simulink model "controller"  (R2025b)
settings: Solver=VariableStepAuto  StartTime=0.0  StopTime=inf  RelTol=1e-3
undefined symbols (not defined in the file): cog_height, DiscIntNeverNeededParam, Fz_stat_FL, Fz_stat_FR, Fz_stat_RL, Fz_stat_RR, lF, lR, pitch_inertia, pitchAngle, pitching_coefficient, pitchStiffness, rdyn, reference_area, rho, rollStiffness_F, rollStiffness_R, sprung_mass, tire, total_pitchDamping, total_pitchStiffness, total_rollStiffness, trackwidth_F, trackwidth_R, unsprung_mass, wheelbase
settings Model: Creator=marce  LastModifiedBy=marce

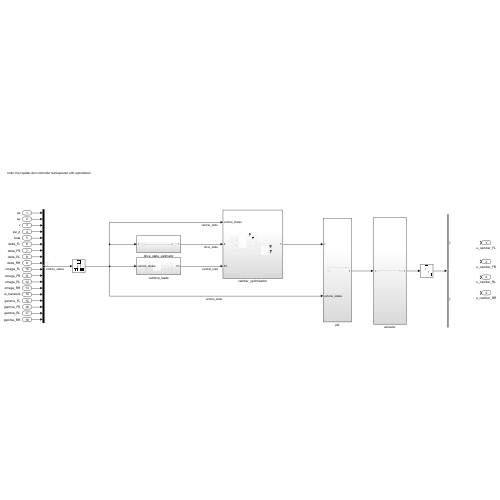
[thumbnail: Simulink's stored preview of the top-level diagram]
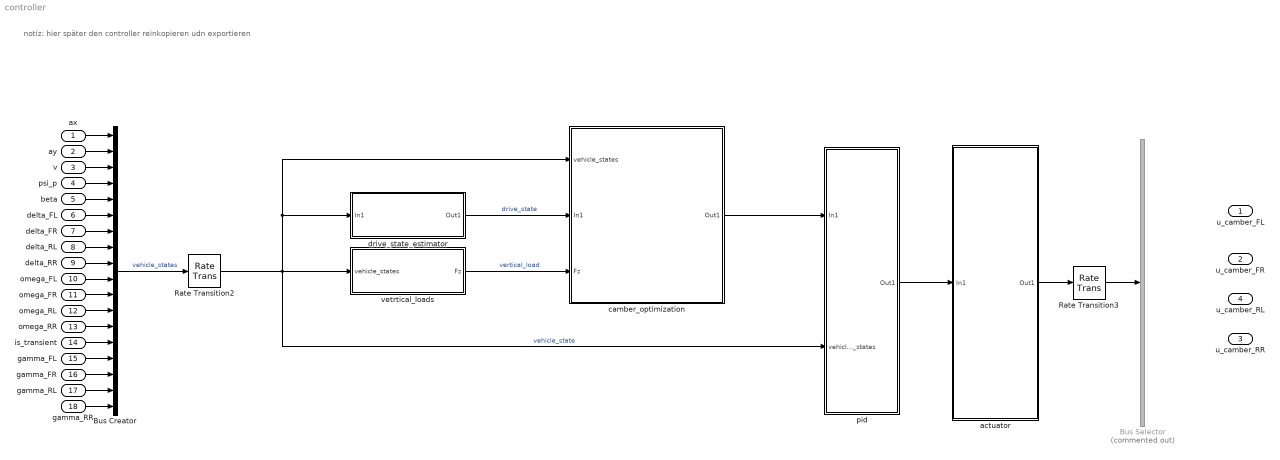
== system controller ==
  note: notiz: hier später den controller reinkopieren udn exportieren
  ax : Inport  OutDataTypeStr=double  Unit=m/s^2
  ay : Inport  Port=2  OutDataTypeStr=double  Unit=m/s^2
  v : Inport  Port=3  OutDataTypeStr=double  Unit=m/s
  psi_p : Inport  Port=4  OutDataTypeStr=double  Unit=rad/s
  beta : Inport  Port=5  OutDataTypeStr=double  Unit=rad
  delta_FL : Inport  Port=6  OutDataTypeStr=double  Unit=rad
  delta_FR : Inport  Port=7  OutDataTypeStr=double  Unit=rad
  delta_RL : Inport  Port=8  OutDataTypeStr=double  Unit=rad
  delta_RR : Inport  Port=9  OutDataTypeStr=double  Unit=rad
  omega_FL : Inport  Port=10  OutDataTypeStr=double  Unit=rad/s
  omega_FR : Inport  Port=11  OutDataTypeStr=double  Unit=rad/s
  omega_RL : Inport  Port=12  OutDataTypeStr=double  Unit=rad/s
  omega_RR : Inport  Port=13  OutDataTypeStr=double  Unit=rad/s
  is_transient : Inport  Port=14  OutDataTypeStr=boolean  Unit=1
  gamma_FL : Inport  Port=15  OutDataTypeStr=double  Unit=rad
  gamma_FR : Inport  Port=16  OutDataTypeStr=double  Unit=rad
  gamma_RL : Inport  Port=17  OutDataTypeStr=double  Unit=rad
  gamma_RR : Inport  Port=18  OutDataTypeStr=double  Unit=rad
  Bus Creator : BusCreator  Inputs=18  OutDataTypeStr=Bus: vehicle_states  NonVirtualBus=on
      settings: InheritFromInputs=off
  Bus Selector : BusSelector  Commented=on  OutputSignals=signal1,signal2
  Rate Transition2 : RateTransition
  Rate Transition3 : RateTransition
  actuator : Subsystem
  camber_optimization : Subsystem
  drive_state_estimator : Subsystem
  pid : Subsystem
  vetrtical_loads : Subsystem
  u_camber_FL : Outport
  u_camber_FR : Outport  Port=2
  u_camber_RR : Outport  Port=3
  u_camber_RL : Outport  Port=4
  wires:
  camber_optimization/1(Out1) -> pid/1(In1)
  Rate Transition2/1 -> camber_optimization/1(vehicle_states), drive_state_estimator/1(In1), vetrtical_loads/1(vehicle_states), pid/2(vehicle_states)  "vehicle_state"
  Rate Transition3/1 -> Bus Selector/1
  pid/1(Out1) -> actuator/1(In1)
  Bus Creator/1 -> Rate Transition2/1  "vehicle_states"
  vetrtical_loads/1(Fz) -> camber_optimization/3(Fz)  "vertical_load"
  drive_state_estimator/1(Out1) -> camber_optimization/2(In1)  "drive_state"
  actuator/1(Out1) -> Rate Transition3/1
  ax/1 -> Bus Creator/1
  ay/1 -> Bus Creator/2
  v/1 -> Bus Creator/3
  psi_p/1 -> Bus Creator/4
  beta/1 -> Bus Creator/5
  delta_FL/1 -> Bus Creator/6
  delta_FR/1 -> Bus Creator/7
  delta_RL/1 -> Bus Creator/8
  delta_RR/1 -> Bus Creator/9
  omega_FL/1 -> Bus Creator/10
  omega_FR/1 -> Bus Creator/11
  omega_RL/1 -> Bus Creator/12
  omega_RR/1 -> Bus Creator/13
  is_transient/1 -> Bus Creator/14
  gamma_FL/1 -> Bus Creator/15
  gamma_FR/1 -> Bus Creator/16
  gamma_RL/1 -> Bus Creator/17
  gamma_RR/1 -> Bus Creator/18

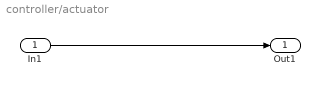
== system controller/actuator ==
  In1 : Inport
  Out1 : Outport
  wires:
  In1/1 -> Out1/1

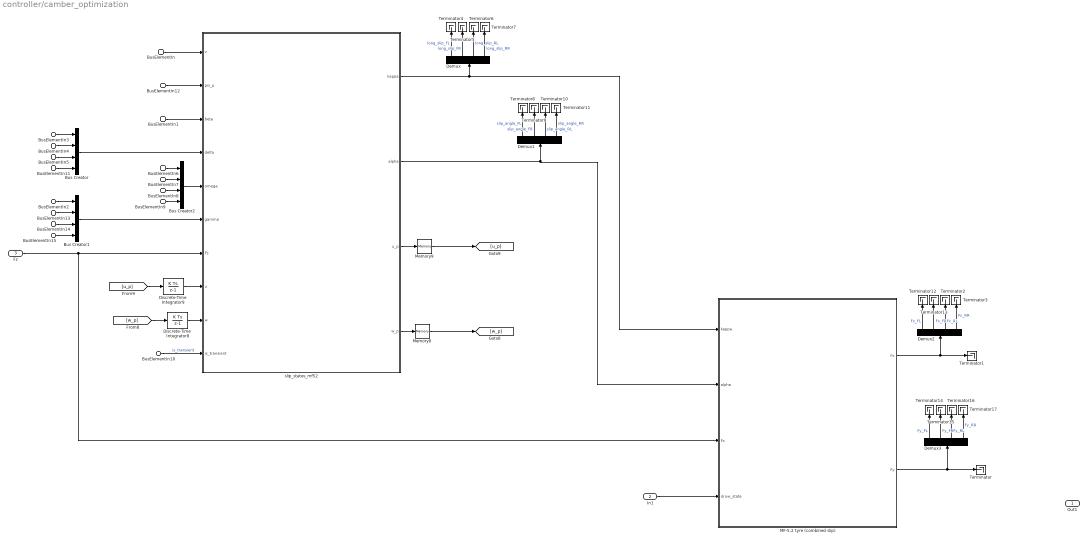
== system controller/camber_optimization ==
  BusElementIn6 : Inport  PortName=vehicle_states  Element=omega_FL
  BusElementIn7 : Inport  PortName=vehicle_states  Element=omega_FR
  BusElementIn8 : Inport  PortName=vehicle_states  Element=omega_RL
  BusElementIn9 : Inport  PortName=vehicle_states  Element=omega_RR
  BusElementIn10 : Inport  PortName=vehicle_states  Element=is_transient
  BusElementIn : Inport  PortName=vehicle_states  Element=v
  BusElementIn3 : Inport  PortName=vehicle_states  Element=delta_FL
  BusElementIn4 : Inport  PortName=vehicle_states  Element=delta_FR
  BusElementIn5 : Inport  PortName=vehicle_states  Element=delta_RL
  BusElementIn11 : Inport  PortName=vehicle_states  Element=delta_RR
  BusElementIn12 : Inport  PortName=vehicle_states  Element=yaw_rate
  BusElementIn1 : Inport  PortName=vehicle_states  Element=side_slip_angle
  BusElementIn2 : Inport  PortName=vehicle_states  Element=camber_FL
  BusElementIn13 : Inport  PortName=vehicle_states  Element=camber_FR
  BusElementIn14 : Inport  PortName=vehicle_states  Element=camber_RL
  BusElementIn15 : Inport  PortName=vehicle_states  Element=camber_RR
  In1 : Inport  Port=2
  Fz : Inport  Port=3
  Bus Creator : BusCreator  Inputs=4
  Bus Creator1 : BusCreator  Inputs=4
  Bus Creator2 : BusCreator  Inputs=4
  Demux{,1..3} (4 alike) : Demux
      settings: DisplayOption=none
  Discrete-Time Integrator8 : DiscreteIntegrator  SampleTime=-1  UpperSaturationLimit=0.1  LowerSaturationLimit=-0.1  ICPrevOutput=DiscIntNeverNeededParam  ICPrevScaledInput=DiscIntNeverNeededParam
  Discrete-Time Integrator9 : DiscreteIntegrator  SampleTime=-1  UpperSaturationLimit=0.01  LowerSaturationLimit=-0.01  ICPrevOutput=DiscIntNeverNeededParam  ICPrevScaledInput=DiscIntNeverNeededParam
  MF-5.2 tyre (combined slip) : MATLAB Function  TreatAsAtomicUnit=on
  Memory8 : Memory
  Memory9 : Memory
  Terminator{,1..17} (18 alike) : Terminator
  slip_states_mf52 : MATLAB Function  TreatAsAtomicUnit=on
  Out1 : Outport
  wires:
  Fz/1 -> slip_states_mf52/7(Fz), MF-5.2 tyre (combined slip)/3(Fz)
  BusElementIn6/1 -> Bus Creator2/1
  BusElementIn7/1 -> Bus Creator2/2
  BusElementIn10/1 -> slip_states_mf52/10(is_transient)  "is_transient"
  BusElementIn8/1 -> Bus Creator2/3
  BusElementIn9/1 -> Bus Creator2/4
  BusElementIn3/1 -> Bus Creator/1
  BusElementIn11/1 -> Bus Creator/4
  BusElementIn5/1 -> Bus Creator/3
  BusElementIn4/1 -> Bus Creator/2
  Bus Creator/1 -> slip_states_mf52/4(delta)
  BusElementIn/1 -> slip_states_mf52/1(v)
  [w_p] -> Discrete-Time Integrator8/1
  Discrete-Time Integrator8/1 -> slip_states_mf52/9(w)
  slip_states_mf52/4(w_p) -> Memory8/1
  Memory8/1 -> [w_p]
  Memory9/1 -> [u_p]
  slip_states_mf52/3(u_p) -> Memory9/1
  [u_p] -> Discrete-Time Integrator9/1
  Discrete-Time Integrator9/1 -> slip_states_mf52/8(u)
  slip_states_mf52/1(kappa) -> MF-5.2 tyre (combined slip)/1(kappa), Demux/1
  slip_states_mf52/2(alpha) -> MF-5.2 tyre (combined slip)/2(alpha), Demux1/1
  BusElementIn12/1 -> slip_states_mf52/2(psi_p)
  BusElementIn1/1 -> slip_states_mf52/3(beta)
  Bus Creator2/1 -> slip_states_mf52/5(omega)
  Demux/1 -> Terminator4/1  "long_slip_FL"
  Demux/2 -> Terminator5/1  "long_slip_FR"
  Demux/3 -> Terminator6/1  "long_slip_RL"
  Demux/4 -> Terminator7/1  "long_slip_RR"
  Demux1/2 -> Terminator9/1  "slip_angle_FR"
  Demux1/1 -> Terminator8/1  "slip_angle_FL"
  Demux1/4 -> Terminator11/1  "slip_angle_RR"
  Demux1/3 -> Terminator10/1  "slip_angle_RL"
  In1/1 -> MF-5.2 tyre (combined slip)/4(drive_state)
  MF-5.2 tyre (combined slip)/1(Fx) -> Demux2/1, Terminator1/1
  MF-5.2 tyre (combined slip)/2(Fy) -> Demux3/1, Terminator/1
  Demux2/2 -> Terminator13/1  "Fx_FR"
  Demux2/4 -> Terminator3/1  "Fx_RR"
  Demux2/3 -> Terminator2/1  "Fx_RL"
  Demux2/1 -> Terminator12/1  "Fx_FL"
  Demux3/3 -> Terminator16/1  "Fy_RL"
  Demux3/4 -> Terminator17/1  "Fy_RR"
  Demux3/1 -> Terminator14/1  "Fy_FL"
  Demux3/2 -> Terminator15/1  "Fy_FR"
  Bus Creator1/1 -> slip_states_mf52/6(gamma)
  BusElementIn2/1 -> Bus Creator1/1
  BusElementIn13/1 -> Bus Creator1/2
  BusElementIn14/1 -> Bus Creator1/3
  BusElementIn15/1 -> Bus Creator1/4

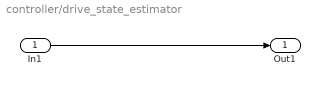
== system controller/drive_state_estimator ==
  In1 : Inport
  Out1 : Outport
  wires:
  In1/1 -> Out1/1

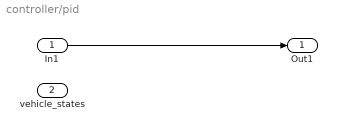
== system controller/pid ==
  In1 : Inport
  vehicle_states : Inport  Port=2
  Out1 : Outport
  wires:
  In1/1 -> Out1/1

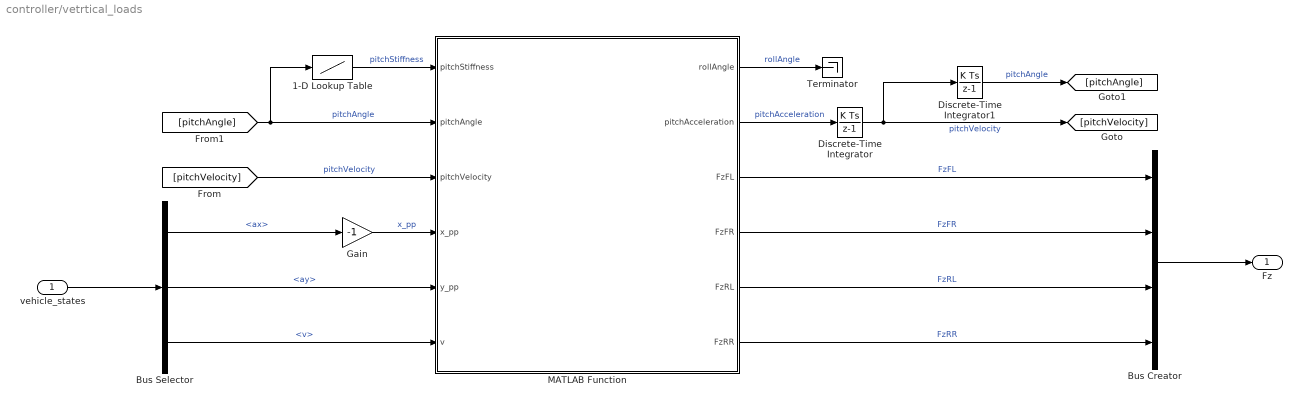
== system controller/vetrtical_loads ==
  vehicle_states : Inport
  1-D Lookup Table : Lookup_n-D  NumberOfTableDimensions=1  BreakpointsForDimension1=pitchAngle  Table=pitchStiffness  InternalRulePriority=Speed  RndMeth=Simplest
  Bus Creator : BusCreator  Inputs=4
  Bus Selector : BusSelector  OutputSignals=ax,ay,v
  Discrete-Time Integrator : DiscreteIntegrator  SampleTime=-1  ICPrevOutput=DiscIntNeverNeededParam  ICPrevScaledInput=DiscIntNeverNeededParam
  Discrete-Time Integrator1 : DiscreteIntegrator  InitialCondition=-0.001  SampleTime=-1  ICPrevOutput=DiscIntNeverNeededParam  ICPrevScaledInput=DiscIntNeverNeededParam
  Gain : Gain  Gain=-1
  MATLAB Function : MATLAB Function  TreatAsAtomicUnit=on
  Terminator : Terminator
  Fz : Outport
  wires:
  MATLAB Function/3(FzFL) -> Bus Creator/1  "FzFL"
  Discrete-Time Integrator1/1 -> [pitchAngle]  "pitchAngle"
  [pitchVelocity] -> MATLAB Function/3(pitchVelocity)  "pitchVelocity"
  Bus Selector/1 -> Gain/1  "<ax>"
  1-D Lookup Table/1 -> MATLAB Function/1(pitchStiffness)  "pitchStiffness"
  MATLAB Function/4(FzFR) -> Bus Creator/2  "FzFR"
  Gain/1 -> MATLAB Function/4(x_pp)  "x_pp"
  MATLAB Function/2(pitchAcceleration) -> Discrete-Time Integrator/1  "pitchAcceleration"
  [pitchAngle] -> 1-D Lookup Table/1, MATLAB Function/2(pitchAngle)  "pitchAngle"
  MATLAB Function/5(FzRL) -> Bus Creator/3  "FzRL"
  MATLAB Function/6(FzRR) -> Bus Creator/4  "FzRR"
  vehicle_states/1 -> Bus Selector/1
  Discrete-Time Integrator/1 -> [pitchVelocity], Discrete-Time Integrator1/1  "pitchVelocity"
  Bus Creator/1 -> Fz/1
  MATLAB Function/1(rollAngle) -> Terminator/1  "rollAngle"
  Bus Selector/2 -> MATLAB Function/5(y_pp)  "<ay>"
  Bus Selector/3 -> MATLAB Function/6(v)  "<v>"

== matlab function controller/vetrtical_loads/MATLAB Function ==
  data: pitchStiffness input; pitchAngle input; pitchVelocity input; x_pp input; rollAngle output; pitchAcceleration output; y_pp input; v input; cog_height parameter; sprung_mass parameter; FzFL output; rollStiffness_F parameter; rollStiffness_R parameter; total_rollStiffness parameter; trackwidth_F parameter; trackwidth_R parameter; Fz_stat_FL parameter; Fz_stat_FR parameter; Fz_stat_RL parameter; Fz_stat_RR parameter; FzFR output; FzRL output; FzRR output; wheelbase parameter; total_pitchStiffness parameter; rdyn parameter; unsprung_mass parameter; pitch_inertia parameter; total_pitchDamping parameter; reference_area parameter; pitching_coefficient parameter; rho parameter
function [rollAngle,pitchAcceleration,FzFL,FzFR,FzRL,FzRR]  = fcn(pitchStiffness,pitchAngle,pitchVelocity,x_pp, y_pp,v, cog_height, sprung_mass,rollStiffness_F,rollStiffness_R,total_rollStiffness,trackwidth_F, trackwidth_R, Fz_stat_FL, Fz_stat_FR, Fz_stat_RL, Fz_stat_RR, wheelbase, total_pitchStiffness, rdyn, unsprung_mass, pitch_inertia, total_pitchDamping, reference_area, pitching_coefficient, rho)

rollTorque = sprung_mass .* y_pp .* cog_height;
rollAngle = rollTorque ./ (total_rollStiffness);

dFz_roll_FL = (rollAngle .* rollStiffness_F - rdyn .* unsprung_mass .* y_pp) ./ trackwidth_F;
dFz_roll_FR = (rollAngle .* rollStiffness_F - rdyn .* unsprung_mass .* y_pp) ./ trackwidth_F;
dFz_roll_RL = (rollAngle .* rollStiffness_R - rdyn .* unsprung_mass .* y_pp) ./ trackwidth_R;
dFz_roll_RR = (rollAngle .* rollStiffness_R - rdyn .* unsprung_mass .* y_pp) ./ trackwidth_R;
           
pitchTorque = sprung_mass .* x_pp .* cog_height - rho ./2 .* pitching_coefficient .* wheelbase .* reference_area .* v^2;
% pitchStiffness = 3.825903e+09 * pitchAngle^3 + -1.854731e+09 * pitchAngle^2 + 1.728035e+08 * pitchAngle + -1.759672e+06;
% pitchStiffness = min(max(pitchStiffness, 290e3), 626e3);
pitchAcceleration = (pitchTorque - total_pitchDamping .* pitchVelocity - pitchStiffness .* pitchAngle) ./ pitch_inertia;

dFz_pitch_FL = (pitchStiffness ./ 2 .* pitchAngle + total_pitchDamping ./ 2 .* pitchVelocity - pitch_inertia ./4 .* pitchAcceleration) ./ wheelbase;
dFz_pitch_FR = (pitchStiffness ./ 2 .* pitchAngle + total_pitchDamping ./ 2 .* pitchVelocity - pitch_inertia ./4 .* pitchAcceleration) ./ wheelbase;
dFz_pitch_RL = (pitchStiffness ./ 2 .* pitchAngle + total_pitchDamping ./ 2 .* pitchVelocity - pitch_inertia ./4 .* pitchAcceleration) ./ wheelbase;
dFz_pitch_RR = (pitchStiffness ./ 2 .* pitchAngle + total_pitchDamping ./ 2 .* pitchVelocity - pitch_inertia ./4 .* pitchAcceleration) ./ wheelbase;

FzFL = Fz_stat_FL + dFz_roll_FL + dFz_pitch_FL;
FzFR = Fz_stat_FR - dFz_roll_FR + dFz_pitch_FR;
FzRL = Fz_stat_RL + dFz_roll_RL - dFz_pitch_RL;
FzRR = Fz_stat_RR - dFz_roll_RR - dFz_pitch_RR;

== matlab function controller/camber_optimization/MF-5.2 tyre (combined slip) ==
  data: kappa input; alpha input; Fz input; drive_state input; Fx output; tire parameter; Fy output
function [Fx, Fy] = fcn(kappa, alpha, Fz, drive_state, tire)
    %% determine output sizes
    % step is needed so simulink now the sizes when compiling
    Fx = zeros(1,4);
    Fy = zeros(1,4);

    %% camber
    gamma_FL = 0; % tyre model needs camber as input wich will be 0 for now
    gamma_FR = 0; % tyre model needs camber as input wich will be 0 for now
    gamma_RL = 0; % tyre model needs camber as input wich will be 0 for now
    gamma_RR = 0; % tyre model needs camber as input wich will be 0 for now

    %% parameter mapping
    % vertical
    F_z0 = tire.Vertical.FNOMIN;

    % longitudinal (pure slip)
    p_Cx1 = tire.Long.PCX1;
    
    p_Dx1 = tire.Long.PDX1;
    p_Dx2 = tire.Long.PDX2;
    p_Dx3 = tire.Long.PDX3;
    
    p_Ex1 = tire.Long.PEX1;
    p_Ex2 = tire.Long.PEX2;
    p_Ex3 = tire.Long.PEX3;
    p_Ex4 = tire.Long.PEX4;
    
    p_Kx1 = tire.Long.PKX1;
    p_Kx2 = tire.Long.PKX2;
    p_Kx3 = tire.Long.PKX3;
    
    p_Hx1 = tire.Long.PHX1;
    p_Hx2 = tire.Long.PHX2;
    
    p_Vx1 = tire.Long.PVX1;
    p_Vx2 = tire.Long.PVX2;
    
    % lateral (pure slip)
    p_Cy1 = tire.Lat.PCY1;
    
    p_Dy1 = tire.Lat.PDY1;
    p_Dy2 = tire.Lat.PDY2;
    p_Dy3 = tire.Lat.PDY3;
    
    p_Ey1 = tire.Lat.PEY1;
    p_Ey2 = tire.Lat.PEY2;
    p_Ey3 = tire.Lat.PEY3;
    p_Ey4 = tire.Lat.PEY4;
    
    p_Ky1 = tire.Lat.PKY1;
    p_Ky2 = tire.Lat.PKY2;
    p_Ky3 = tire.Lat.PKY3;
    
    p_Hy1 = tire.Lat.PHY1;
    p_Hy2 = tire.Lat.PHY2;
    p_Hy3 = tire.Lat.PHY3;
    
    p_Vy1 = tire.Lat.PVY1;
    p_Vy2 = tire.Lat.PVY2;
    p_Vy3 = tire.Lat.PVY3;
    p_Vy4 = tire.Lat.PVY4;
    
    % longitudinal (combined slip)
    r_Bx1 = tire.Long.RBX1;
    r_Bx2 = tire.Long.RBX2;
    
    r_Cx1 = tire.Long.RCX1;
    
    r_Ex1 = tire.Long.REX1;
    r_Ex2 = tire.Long.REX2;
    
    r_Hx1 = tire.Long.RHX1;
    
    % lateral (combined slip)
    r_By1 = tire.Lat.RBY1;
    r_By2 = tire.Lat.RBY2;
    r_By3 = tire.Lat.RBY3;
    
    r_Cy1 = tire.Lat.RCY1;
    
    r_Ey1 = tire.Lat.REY1;
    r_Ey2 = tire.Lat.REY2;
    
    r_Hy1 = tire.Lat.RHY1;
    r_Hy2 = tire.Lat.RHY2;
    
    r_Vy1 = tire.Lat.RVY1;
    r_Vy2 = tire.Lat.RVY2;
    r_Vy3 = tire.Lat.RVY3;
    r_Vy4 = tire.Lat.RVY4;
    r_Vy5 = tire.Lat.RVY5;
    r_Vy6 = tire.Lat.RVY6;

    %% vertical load mapping
    Fz_FL = Fz(1);
    Fz_FR = Fz(2);
    Fz_RL = Fz(3);
    Fz_RR = Fz(4);

    %% longitudinal slip mapping
    long_slip_FL = kappa(1);
    long_slip_FR = kappa(2);
    long_slip_RL = kappa(3);
    long_slip_RR = kappa(4);

    %% side slip angle mapping
    slip_ang_FL = alpha(1);
    slip_ang_FR = alpha(2);
    slip_ang_RL = alpha(3);
    slip_ang_RR = alpha(4);

    %% normalized vertical load
    % equations from Delft MF-Tyre User Manual Version 5.2
    % page 17
    dfz_FL = (Fz_FL - F_z0) / F_z0;
    dfz_FR = (Fz_FR - F_z0) / F_z0; 
    dfz_RL = (Fz_RL - F_z0) / F_z0; 
    dfz_RR = (Fz_RR - F_z0) / F_z0;

    %% longitudinal (pure slip)
    % equations from Delft MF-Tyre User Manual Version 5.2
    % page 22 - 24
    Cx = p_Cx1; % - each wheel is equipped with the same tyre
    
    mu_x_FL = (p_Dx1 + p_Dx2 .* dfz_FL) .* (1 - p_Dx3 .* gamma_FL.^2);
    mu_x_FR = (p_Dx1 + p_Dx2 .* dfz_FR) .* (1 - p_Dx3 .* gamma_FR.^2);
    mu_x_RL = (p_Dx1 + p_Dx2 .* dfz_RL) .* (1 - p_Dx3 .* gamma_RL.^2);
    mu_x_RR = (p_Dx1 + p_Dx2 .* dfz_RR) .* (1 - p_Dx3 .* gamma_RR.^2);

    Dx_FL = mu_x_FL .* Fz_FL;
    Dx_FR = mu_x_FR .* Fz_FR;
    Dx_RL = mu_x_RL .* Fz_RL;
    Dx_RR = mu_x_RR .* Fz_RR;
    
    S_Hx_FL = (p_Hx1 + p_Hx2 .* dfz_FL);
    S_Hx_FR = (p_Hx1 + p_Hx2 .* dfz_FR);
    S_Hx_RL = (p_Hx1 + p_Hx2 .* dfz_RL);
    S_Hx_RR = (p_Hx1 + p_Hx2 .* dfz_RR);

    S_Vx_FL = Fz_FL .* (p_Vx1 + p_Vx2 .* dfz_FL);
    S_Vx_FR = Fz_FR .* (p_Vx1 + p_Vx2 .* dfz_FR);
    S_Vx_RL = Fz_RL .* (p_Vx1 + p_Vx2 .* dfz_RL);
    S_Vx_RR = Fz_RR .* (p_Vx1 + p_Vx2 .* dfz_RR);
    
    kappa_x_FL = long_slip_FL + S_Hx_FL;
    kappa_x_FR = long_slip_FR + S_Hx_FR;
    kappa_x_RL = long_slip_RL + S_Hx_RL;
    kappa_x_RR = long_slip_RR + S_Hx_RR;
    
    Ex_FL = (p_Ex1 + p_Ex2 .* dfz_FL + p_Ex3 .* dfz_FL.^2) .* (1 - p_Ex4 .* sign(kappa_x_FL));
    Ex_FR = (p_Ex1 + p_Ex2 .* dfz_FR + p_Ex3 .* dfz_FR.^2) .* (1 - p_Ex4 .* sign(kappa_x_FR));
    Ex_RL = (p_Ex1 + p_Ex2 .* dfz_RL + p_Ex3 .* dfz_RL.^2) .* (1 - p_Ex4 .* sign(kappa_x_RL));
    Ex_RR = (p_Ex1 + p_Ex2 .* dfz_RR + p_Ex3 .* dfz_RR.^2) .* (1 - p_Ex4 .* sign(kappa_x_RR));

    Kx_FL = Fz_FL .* (p_Kx1 + p_Kx2 .* dfz_FL) .* exp(p_Kx3 .* dfz_FL);
    Kx_FR = Fz_FR .* (p_Kx1 + p_Kx2 .* dfz_FR) .* exp(p_Kx3 .* dfz_FR);
    Kx_RL = Fz_RL .* (p_Kx1 + p_Kx2 .* dfz_RL) .* exp(p_Kx3 .* dfz_RL);
    Kx_RR = Fz_RR .* (p_Kx1 + p_Kx2 .* dfz_RR) .* exp(p_Kx3 .* dfz_RR);

    Bx_FL = Kx_FL ./ (Cx .* Dx_FL);
    Bx_FR = Kx_FR ./ (Cx .* Dx_FR);
    Bx_RL = Kx_RL ./ (Cx .* Dx_RL);
    Bx_RR = Kx_RR ./ (Cx .* Dx_RR);
    
    Fx0_FL = Dx_FL .* sin(Cx .* atan(Bx_FL .* kappa_x_FL - Ex_FL .* (Bx_FL .* kappa_x_FL - atan(Bx_FL .* kappa_x_FL)))) + S_Vx_FL; % will later be used in combined slip equations
    Fx0_FR = Dx_FR .* sin(Cx .* atan(Bx_FR .* kappa_x_FR - Ex_FR .* (Bx_FR .* kappa_x_FR - atan(Bx_FR .* kappa_x_FR)))) + S_Vx_FR; % will later be used in combined slip equations
    Fx0_RL = Dx_RL .* sin(Cx .* atan(Bx_RL .* kappa_x_RL - Ex_RL .* (Bx_RL .* kappa_x_RL - atan(Bx_RL .* kappa_x_RL)))) + S_Vx_RL; % will later be used in combined slip equations
    Fx0_RR = Dx_RR .* sin(Cx .* atan(Bx_RR .* kappa_x_RR - Ex_RR .* (Bx_RR .* kappa_x_RR - atan(Bx_RR .* kappa_x_RR)))) + S_Vx_RR; % will later be used in combined slip equations

    %% lateral (pure slip)
    % equations from Delft MF-Tyre User Manual Version 5.2
    % page 24 - 26
    Cy = p_Cy1;

    mu_y_FL = (p_Dy1 + p_Dy2 .* dfz_FL) .* (1-p_Dy3 .* gamma_FL.^2);
    mu_y_FR = (p_Dy1 + p_Dy2 .* dfz_FR) .* (1-p_Dy3 .* gamma_FR.^2);
    mu_y_RL = (p_Dy1 + p_Dy2 .* dfz_RL) .* (1-p_Dy3 .* gamma_RL.^2);
    mu_y_RR = (p_Dy1 + p_Dy2 .* dfz_RR) .* (1-p_Dy3 .* gamma_RR.^2);

    Dy_FL = mu_y_FL .* Fz_FL;
    Dy_FR = mu_y_FR .* Fz_FR;
    Dy_RL = mu_y_RL .* Fz_RL;
    Dy_RR = mu_y_RR .* Fz_RR;
    
    S_Hy_FL = p_Hy1 + p_Hy2 .* dfz_FL + p_Hy3 .* gamma_FL;
    S_Hy_FR = p_Hy1 + p_Hy2 .* dfz_FR + p_Hy3 .* gamma_FR;
    S_Hy_RL = p_Hy1 + p_Hy2 .* dfz_RL + p_Hy3 .* gamma_RL;
    S_Hy_RR = p_Hy1 + p_Hy2 .* dfz_RR + p_Hy3 .* gamma_RR;

    S_Vy_FL = Fz_FL .* (p_Vy1 + p_Vy2 .* dfz_FL + (p_Vy3 + p_Vy4 .* dfz_FL) .* gamma_FL);
    S_Vy_FR = Fz_FR .* (p_Vy1 + p_Vy2 .* dfz_FR + (p_Vy3 + p_Vy4 .* dfz_FR) .* gamma_FR);
    S_Vy_RL = Fz_RL .* (p_Vy1 + p_Vy2 .* dfz_RL + (p_Vy3 + p_Vy4 .* dfz_RL) .* gamma_RL);
    S_Vy_RR = Fz_RR .* (p_Vy1 + p_Vy2 .* dfz_RR + (p_Vy3 + p_Vy4 .* dfz_RR) .* gamma_RR);
    
    alpha_y_FL = slip_ang_FL + S_Hy_FL;
    alpha_y_FR = slip_ang_FR + S_Hy_FR;
    alpha_y_RL = slip_ang_RL + S_Hy_RL;
    alpha_y_RR = slip_ang_RR + S_Hy_RR;
    
    Ey_FL = (p_Ey1 + p_Ey2 .* dfz_FL) .* (1 - (p_Ey3 + p_Ey4 .* gamma_FL) .* sign(alpha_y_FL));
    Ey_FR = (p_Ey1 + p_Ey2 .* dfz_FR) .* (1 - (p_Ey3 + p_Ey4 .* gamma_FR) .* sign(alpha_y_FR));
    Ey_RL = (p_Ey1 + p_Ey2 .* dfz_RL) .* (1 - (p_Ey3 + p_Ey4 .* gamma_RL) .* sign(alpha_y_RL));
    Ey_RR = (p_Ey1 + p_Ey2 .* dfz_RR) .* (1 - (p_Ey3 + p_Ey4 .* gamma_RR) .* sign(alpha_y_RR));

    Ky_FL = p_Ky1 .* F_z0 .* sin(2 .* atan(Fz_FL ./ (p_Ky2 .* F_z0))) .* (1 - p_Ky3 .* abs(gamma_FL));
    Ky_FR = p_Ky1 .* F_z0 .* sin(2 .* atan(Fz_FR ./ (p_Ky2 .* F_z0))) .* (1 - p_Ky3 .* abs(gamma_FR));
    Ky_RL = p_Ky1 .* F_z0 .* sin(2 .* atan(Fz_RL ./ (p_Ky2 .* F_z0))) .* (1 - p_Ky3 .* abs(gamma_RL));
    Ky_RR = p_Ky1 .* F_z0 .* sin(2 .* atan(Fz_RR ./ (p_Ky2 .* F_z0))) .* (1 - p_Ky3 .* abs(gamma_RR));

    By_FL = Ky_FL / (Cy .* Dy_FL);
    By_FR = Ky_FR / (Cy .* Dy_FR);
    By_RL = Ky_RL / (Cy .* Dy_RL);
    By_RR = Ky_RR / (Cy .* Dy_RR);
    
    Fy0_FL = Dy_FL .* sin(Cy .* atan(By_FL .* alpha_y_FL - Ey_FL .* (By_FL .* alpha_y_FL - atan(By_FL .* alpha_y_FL)))) + S_Vy_FL; % will later be used in combined slip equations 
    Fy0_FR = Dy_FR .* sin(Cy .* atan(By_FR .* alpha_y_FR - Ey_FR .* (By_FR .* alpha_y_FR - atan(By_FR .* alpha_y_FR)))) + S_Vy_FR; % will later be used in combined slip equations 
    Fy0_RL = Dy_RL .* sin(Cy .* atan(By_RL .* alpha_y_RL - Ey_RL .* (By_RL .* alpha_y_RL - atan(By_RL .* alpha_y_RL)))) + S_Vy_RL; % will later be used in combined slip equations 
    Fy0_RR = Dy_RR .* sin(Cy .* atan(By_RR .* alpha_y_RR - Ey_RR .* (By_RR .* alpha_y_RR - atan(By_RR .* alpha_y_RR)))) + S_Vy_RR; % will later be used in combined slip equations 

    %% longitudinal (combined slip)
    % equations from Delft MF-Tyre User Manual Version 5.2
    % page 30 - 31
    S_Hxa = r_Hx1;

    alpha_s_FL = slip_ang_FL + S_Hxa;
    alpha_s_FR = slip_ang_FR + S_Hxa;
    alpha_s_RL = slip_ang_RL + S_Hxa;
    alpha_s_RR = slip_ang_RR + S_Hxa;
    
    Bxa_FL = r_Bx1 .* cos(atan(r_Bx2 .* long_slip_FL));
    Bxa_FR = r_Bx1 .* cos(atan(r_Bx2 .* long_slip_FR));
    Bxa_RL = r_Bx1 .* cos(atan(r_Bx2 .* long_slip_RL));
    Bxa_RR = r_Bx1 .* cos(atan(r_Bx2 .* long_slip_RR));

    Cxa = r_Cx1;

    Exa_FL = r_Ex1 + r_Ex2 .* dfz_FL;
    Exa_FR = r_Ex1 + r_Ex2 .* dfz_FR;
    Exa_RL = r_Ex1 + r_Ex2 .* dfz_RL;
    Exa_RR = r_Ex1 + r_Ex2 .* dfz_RR;
    
    Gxa_FL = (cos(Cxa .* atan(Bxa_FL .* alpha_s_FL - Exa_FL .* (Bxa_FL .* alpha_s_FL - atan(Bxa_FL .* alpha_s_FL))))) ./ ...
        (cos(Cxa .* atan(Bxa_FL .* S_Hxa - Exa_FL .* (Bxa_FL .* S_Hxa - atan(Bxa_FL .* S_Hxa)))));

    Gxa_FR = (cos(Cxa .* atan(Bxa_FR .* alpha_s_FR - Exa_FR .* (Bxa_FR .* alpha_s_FR - atan(Bxa_FR .* alpha_s_FR))))) ./ ...
        (cos(Cxa .* atan(Bxa_FR .* S_Hxa - Exa_FR .* (Bxa_FR .* S_Hxa - atan(Bxa_FR .* S_Hxa)))));
    
    Gxa_RL = (cos(Cxa .* atan(Bxa_RL .* alpha_s_RL - Exa_RL .* (Bxa_RL .* alpha_s_RL - atan(Bxa_RL .* alpha_s_RL))))) ./ ...
        (cos(Cxa .* atan(Bxa_RL .* S_Hxa - Exa_RL .* (Bxa_RL .* S_Hxa - atan(Bxa_RL .* S_Hxa)))));

    Gxa_RR = (cos(Cxa .* atan(Bxa_RR .* alpha_s_RR - Exa_RR .* (Bxa_RR .* alpha_s_RR - atan(Bxa_RR .* alpha_s_RR))))) ./ ...
        (cos(Cxa .* atan(Bxa_RR .* S_Hxa - Exa_RR .* (Bxa_RR .* S_Hxa - atan(Bxa_RR .* S_Hxa)))));
    
    Fx_FL = Fx0_FL .* Gxa_FL;
    Fx_FR = Fx0_FR .* Gxa_FR;
    Fx_RL = Fx0_RL .* Gxa_RL;
    Fx_RR = Fx0_RR .* Gxa_RR;

    %% lateral (combined slip)
    % equations from Delft MF-Tyre User Manual Version 5.2
    % page 32 - 33
    S_Hyk_FL = r_Hy1 + r_Hy2 .* dfz_FL;
    S_Hyk_FR = r_Hy1 + r_Hy2 .* dfz_FR;
    S_Hyk_RL = r_Hy1 + r_Hy2 .* dfz_RL;
    S_Hyk_RR = r_Hy1 + r_Hy2 .* dfz_RR;

    kappa_s_FL = long_slip_FL + S_Hyk_FL;
    kappa_s_FR = long_slip_FR + S_Hyk_FR;
    kappa_s_RL = long_slip_RL + S_Hyk_RL;
    kappa_s_RR = long_slip_RR + S_Hyk_RR;
    
    Byk_FL = r_By1 .* cos(atan(r_By2 .* (slip_ang_FL - r_By3)));
    Byk_FR = r_By1 .* cos(atan(r_By2 .* (slip_ang_FR - r_By3)));
    Byk_RL = r_By1 .* cos(atan(r_By2 .* (slip_ang_RL - r_By3)));
    Byk_RR = r_By1 .* cos(atan(r_By2 .* (slip_ang_RR - r_By3)));

    Cyk = r_Cy1;

    Eyk_FL = r_Ey1 + r_Ey2 .* dfz_FL;
    Eyk_FR = r_Ey1 + r_Ey2 .* dfz_FR;
    Eyk_RL = r_Ey1 + r_Ey2 .* dfz_RL;
    Eyk_RR = r_Ey1 + r_Ey2 .* dfz_RR;
    
    D_Vyk_FL = mu_y_FL .* Fz_FL .* (r_Vy1 + r_Vy2 .* dfz_FL + r_Vy3 .* gamma_FL) .* cos(atan(r_Vy4 .* slip_ang_FL));
    D_Vyk_FR = mu_y_FR .* Fz_FR .* (r_Vy1 + r_Vy2 .* dfz_FR + r_Vy3 .* gamma_FR) .* cos(atan(r_Vy4 .* slip_ang_FR));
    D_Vyk_RL = mu_y_RL .* Fz_RL .* (r_Vy1 + r_Vy2 .* dfz_RL + r_Vy3 .* gamma_RL) .* cos(atan(r_Vy4 .* slip_ang_RL));
    D_Vyk_RR = mu_y_RR .* Fz_RR .* (r_Vy1 + r_Vy2 .* dfz_RR + r_Vy3 .* gamma_RR) .* cos(atan(r_Vy4 .* slip_ang_RR));

    S_Vyk_FL = D_Vyk_FL .* sin(r_Vy5 .* atan(r_Vy6 .* long_slip_FL));
    S_Vyk_FR = D_Vyk_FR .* sin(r_Vy5 .* atan(r_Vy6 .* long_slip_FR));
    S_Vyk_RL = D_Vyk_RL .* sin(r_Vy5 .* atan(r_Vy6 .* long_slip_RL));
    S_Vyk_RR = D_Vyk_RR .* sin(r_Vy5 .* atan(r_Vy6 .* long_slip_RR));
    
    Gyk_FL = (cos(Cyk .* atan(Byk_FL .* kappa_s_FL - Eyk_FL .* (Byk_FL .* kappa_s_FL - atan(Byk_FL .* kappa_s_FL))))) ./ ...
        (cos(Cyk .* atan(Byk_FL .* S_Hyk_FL - Eyk_FL .* (Byk_FL .* S_Hyk_FL - atan(Byk_FL .* S_Hyk_FL)))));

    Gyk_FR = (cos(Cyk .* atan(Byk_FR .* kappa_s_FR - Eyk_FR .* (Byk_FR .* kappa_s_FR - atan(Byk_FR .* kappa_s_FR))))) ./ ...
        (cos(Cyk .* atan(Byk_FR .* S_Hyk_FR - Eyk_FR .* (Byk_FR .* S_Hyk_FR - atan(Byk_FR .* S_Hyk_FR)))));
    
    Gyk_RL = (cos(Cyk .* atan(Byk_RL .* kappa_s_RL - Eyk_RL .* (Byk_RL .* kappa_s_RL - atan(Byk_RL .* kappa_s_RL))))) ./ ...
        (cos(Cyk .* atan(Byk_RL .* S_Hyk_RL - Eyk_RL .* (Byk_RL .* S_Hyk_RL - atan(Byk_RL .* S_Hyk_RL)))));
    
    Gyk_RR = (cos(Cyk .* atan(Byk_RR .* kappa_s_RR - Eyk_RR .* (Byk_RR .* kappa_s_RR - atan(Byk_RR .* kappa_s_RR))))) ./ ...
        (cos(Cyk .* atan(Byk_RR .* S_Hyk_RR - Eyk_RR .* (Byk_RR .* S_Hyk_RR - atan(Byk_RR .* S_Hyk_RR)))));
    
    Fy_FL = Fy0_FL .* Gyk_FL + S_Vyk_FL; if isnan(Fy_FL); Fy_FL = 0; end
    Fy_FR = Fy0_FR .* Gyk_FR + S_Vyk_FR; if isnan(Fy_FR); Fy_FR = 0; end
    Fy_RL = Fy0_RL .* Gyk_RL + S_Vyk_RL; if isnan(Fy_RL); Fy_RL = 0; end
    Fy_RR = Fy0_RR .* Gyk_RR + S_Vyk_RR; if isnan(Fy_RR); Fy_RR = 0; end

    %% outputs
    Fx = [Fx_FL, Fx_FR, Fx_RL, Fx_RR];
    Fy = [Fy_FL, Fy_FR, Fy_RL, Fy_RR];

== matlab function controller/camber_optimization/slip_states_mf52 ==
  data: v input; kappa output; psi_p input; beta input; delta input; omega input; gamma input; Fz input; u input; w input; is_transient input; alpha output; tire parameter; u_p output; w_p output; lF parameter; lR parameter; trackwidth_R parameter; trackwidth_F parameter
function [kappa, alpha, u_p, w_p]= fcn(v, psi_p, beta, delta, omega, gamma, Fz, u, w, is_transient, tire, lF, lR, trackwidth_R, trackwidth_F)
    %% determine output sizes
    % step is needed so simulink now the sizes when compiling
    kappa = zeros(1,4);
    alpha = zeros(1,4);
    u_p   = zeros(1,4);
    w_p   = zeros(1,4);    
           
    %% parameters
    % vertical
    F_z0 = tire.Vertical.FNOMIN;
    c_z = tire.Vertical.VERTICAL_STIFFNESS;
    
    b_reff = tire.Vertical.BREFF;
    d_reff = tire.Vertical.DREFF;
    f_reff = tire.Vertical.FREFF;

    % dimension
    r_0 = tire.Dim.UNLOADED_RADIUS;

    % longitudinal (transient)
    p_Tx1 = tire.Long.PTX1;
    p_Tx2 = tire.Long.PTX2;
    p_Tx3 = tire.Long.PTX3;

    % lateral (transient)
    p_Ty1 = tire.Lat.PTY1;
    p_Ty2 = tire.Lat.PTY2;

    % lateral (pure slip)
    p_Ky3 = tire.Lat.PKY3;

    %% wheel steering angle mapping
    delta_FL = delta(1);
    delta_FR = delta(2);
    delta_RL = delta(3);
    delta_RR = delta(4);

    %% wheel rotational velocity mapping
    omega_FL = omega(1);
    omega_FR = omega(2);
    omega_RL = omega(3);
    omega_RR = omega(4);

    %% current camber mapping
    gamma_FL = gamma(1);
    gamma_FR = gamma(2);
    gamma_RL = gamma(3);
    gamma_RR = gamma(4);

    %% vertical load mapping
    Fz_FL = Fz(1);
    Fz_FR = Fz(2);
    Fz_RL = Fz(3);
    Fz_RR = Fz(4);

    %% longitudinal tyre deflection mapping
    u_FL = min(max(u(1), -0.01), 0.01);
    u_FR = min(max(u(2), -0.01), 0.01);
    u_RL = u(3);
    u_RR = u(4);

    %% lateral tyre deflection mapping
    w_FL = w(1);
    w_FR = w(2);
    w_RL = w(3);
    w_RR = w(4);

    %% effective rolling radius r_e
    % equations from Delft MF-Tyre User Manual Version 5.2
    % page 9 - 11
    p_FL = Fz_FL ./ c_z;
    p_FR = Fz_FR ./ c_z;
    p_RL = Fz_RL ./ c_z;
    p_RR = Fz_RR ./ c_z;
    
    p_Fz0 = F_z0 ./ c_z;
    
    p_d_FL = p_FL ./ p_Fz0;
    p_d_FR = p_FR ./ p_Fz0;
    p_d_RL = p_RL ./ p_Fz0;
    p_d_RR = p_RR ./ p_Fz0;
    
    r_e_FL = r_0 - (p_Fz0 .* (f_reff .* p_d_FL + d_reff .* atan(b_reff .* p_d_FL)));
    r_e_FR = r_0 - (p_Fz0 .* (f_reff .* p_d_FR + d_reff .* atan(b_reff .* p_d_FR)));
    r_e_RL = r_0 - (p_Fz0 .* (f_reff .* p_d_RL + d_reff .* atan(b_reff .* p_d_RL)));
    r_e_RR = r_0 - (p_Fz0 .* (f_reff .* p_d_RR + d_reff .* atan(b_reff .* p_d_RR)));
    
    %% velocity states
    % equation herritage not clear
    v_xFL = v .* cos(beta) - psi_p .* (trackwidth_F ./ 2);
    v_xFR = v .* cos(beta) + psi_p .* (trackwidth_F ./ 2);
    v_xRL = v .* cos(beta) - psi_p .* (trackwidth_R ./ 2);
    v_xRR = v .* cos(beta) + psi_p .* (trackwidth_F ./ 2);
    
    v_yFL = v .* sin(beta) + psi_p .* lF;
    v_yFR = v .* sin(beta) + psi_p .* lF;
    v_yRL = v .* sin(beta) - psi_p .* lR;
    v_yRR = v .* sin(beta) - psi_p .* lR;
    
    % vx in tire coordinate system 
    v_lon_FL = v_xFL .* cos(delta_FL) + v_yFL .* sin(delta_FL);
    v_lon_FR = v_xFR .* cos(delta_FR) + v_yFR .* sin(delta_FR);
    v_lon_RL = v_xRL .* cos(delta_RL) + v_yRL .* sin(delta_RL);
    v_lon_RR = v_xRR .* cos(delta_RR) + v_yRR .* sin(delta_RR);
    
    v_lat_FL = v_xFL .* sin(delta_FL) - v_yFL .* cos(delta_FL);
    v_lat_FR = v_xFR .* sin(delta_FR) - v_yFR .* cos(delta_FR);
    v_lat_RL = v_xRL .* sin(delta_RL) - v_yRL .* cos(delta_RL);
    v_lat_RR = v_xRR .* sin(delta_RR) - v_yRR .* cos(delta_RR);
    
    %% normalized vertical load
    % equations from Delft MF-Tyre User Manual Version 5.2
    % page 17
    dfz_FL = (Fz_FL - F_z0) ./ F_z0;
    dfz_FR = (Fz_FR - F_z0) ./ F_z0; 
    dfz_RL = (Fz_RL - F_z0) ./ F_z0; 
    dfz_RR = (Fz_RR - F_z0) ./ F_z0;
    
    %% longitudinal slip - kappa
    % equations from Delft MF-Tyre User Manual Version 5.2
    % page 12
    v_sx_FL = v_lon_FL - omega_FL .* r_e_FL;
    v_sx_FR = v_lon_FR - omega_FR .* r_e_FR;
    v_sx_RL = v_lon_RL - omega_RL .* r_e_RL;
    v_sx_RR = v_lon_RR - omega_RR .* r_e_RR;

    if is_transient
        % relaxation length
        sigma_k_FL = Fz_FL .* (p_Tx1 + p_Tx2 .* dfz_FL) .* exp(-p_Tx3 .* dfz_FL) .* (r_0 ./ F_z0);
        sigma_k_FR = Fz_FR .* (p_Tx1 + p_Tx2 .* dfz_FR) .* exp(-p_Tx3 .* dfz_FR) .* (r_0 ./ F_z0);
        sigma_k_RL = Fz_RL .* (p_Tx1 + p_Tx2 .* dfz_RL) .* exp(-p_Tx3 .* dfz_RL) .* (r_0 ./ F_z0);
        sigma_k_RR = Fz_RR .* (p_Tx1 + p_Tx2 .* dfz_RR) .* exp(-p_Tx3 .* dfz_RR) .* (r_0 ./ F_z0);

        u_p_FL = -v_sx_FL - (abs(v_lon_FL) ./ sigma_k_FL) .* u_FL;
        u_p_FR = -v_sx_FR - (abs(v_lon_FR) ./ sigma_k_FR) .* u_FR;
        u_p_RL = -v_sx_RL - (abs(v_lon_RL) ./ sigma_k_RL) .* u_RL;
        u_p_RR = -v_sx_RR - (abs(v_lon_RR) ./ sigma_k_RR) .* u_RR;

        long_slip_FL = (u_FL ./ sigma_k_FL) .* sign(v_lon_FL); if isnan(long_slip_FL); long_slip_FL = - v_sx_FL ./ v_lon_FL; end % switch to non transient if Fz not defined
        long_slip_FR = (u_FR ./ sigma_k_FR) .* sign(v_lon_FR); if isnan(long_slip_FR); long_slip_FR = - v_sx_FR ./ v_lon_FR; end % switch to non transient if Fz not defined
        long_slip_RL = (u_RL ./ sigma_k_RL) .* sign(v_lon_RL); if isnan(long_slip_RL); long_slip_RL = - v_sx_RL ./ v_lon_RL; end % switch to non transient if Fz not defined
        long_slip_RR = (u_RR ./ sigma_k_RR) .* sign(v_lon_RR); if isnan(long_slip_RR); long_slip_RR = - v_sx_RR ./ v_lon_RR; end % switch to non transient if Fz not defined
    else
        long_slip_FL = - v_sx_FL ./ v_lon_FL;
        long_slip_FR = - v_sx_FR ./ v_lon_FR;
        long_slip_RL = - v_sx_RL ./ v_lon_RL;
        long_slip_RR = - v_sx_RR ./ v_lon_RR;

        u_p_FL = 0;
        u_p_FR = 0;
        u_p_RL = 0;
        u_p_RR = 0;
    end

    %% slip angle - alpha
    % effektiver Lenkwinkel
    delta_eff_FL = atan(v_yFL ./ v_xFL);
    delta_eff_FR = atan(v_yFR ./ v_xFR);
    delta_eff_RL = atan(v_yRL ./ v_xRL);
    delta_eff_RR = atan(v_yRR ./ v_xRR);
    
    if is_transient
        sigma_a_FL = p_Ty1 .* sin(2.*atan(Fz_FL ./ (p_Ty2 .* F_z0))) .* (1 - p_Ky3 .* abs(gamma_FL)) .* r_0;
        sigma_a_FR = p_Ty1 .* sin(2.*atan(Fz_FR ./ (p_Ty2 .* F_z0))) .* (1 - p_Ky3 .* abs(gamma_FR)) .* r_0;
        sigma_a_RL = p_Ty1 .* sin(2.*atan(Fz_RL ./ (p_Ty2 .* F_z0))) .* (1 - p_Ky3 .* abs(gamma_RL)) .* r_0;
        sigma_a_RR = p_Ty1 .* sin(2.*atan(Fz_RR ./ (p_Ty2 .* F_z0))) .* (1 - p_Ky3 .* abs(gamma_RR)) .* r_0;

        w_p_FL = v_lat_FL - (abs(v_lon_FL) ./ sigma_a_FL) .* w_FL;
        w_p_FR = v_lat_FR - (abs(v_lon_FR) ./ sigma_a_FR) .* w_FR;
        w_p_RL = v_lat_RL - (abs(v_lon_RL) ./ sigma_a_RL) .* w_RL;
        w_p_RR = v_lat_RR - (abs(v_lon_RR) ./ sigma_a_RR) .* w_RR;

        slip_ang_FL = -atan(w_FL ./ sigma_a_FL); % if isnan(slip_ang_FL); slip_ang_FL = -(delta_FL - delta_eff_FL); end % switch to non transient if Fz not defined
        slip_ang_FR = -atan(w_FR ./ sigma_a_FR); % if isnan(slip_ang_FR); slip_ang_FR = -(delta_FR - delta_eff_FR); end % switch to non transient if Fz not defined
        slip_ang_RL = -atan(w_RL ./ sigma_a_RL); % if isnan(slip_ang_RL); slip_ang_RL = -(delta_RL - delta_eff_RL); end % switch to non transient if Fz not defined
        slip_ang_RR = -atan(w_RR ./ sigma_a_RR); % if isnan(slip_ang_RR); slip_ang_RR = -(delta_RR - delta_eff_RR); end % switch to non transient if Fz not defined

    else
        slip_ang_FL = -(delta_FL - delta_eff_FL);
        slip_ang_FR = -(delta_FR - delta_eff_FR);
        slip_ang_RL = -(delta_RL - delta_eff_RL);
        slip_ang_RR = -(delta_RR - delta_eff_RR);

        w_p_FL = 0;
        w_p_FR = 0;
        w_p_RL = 0;
        w_p_RR = 0;
    end

    %% outputs
    kappa = [long_slip_FL, long_slip_FR, long_slip_RL, long_slip_RR];
    alpha = [slip_ang_FL, slip_ang_FR, slip_ang_RL, slip_ang_RR];
    
    u_p   = [u_p_FL, u_p_FR, u_p_RL, u_p_RR];
    w_p   = [w_p_FL, w_p_FR, w_p_RL, w_p_RR];
